simulink model "spwm"  (R2023b)
settings: Solver=VariableStepAuto  StartTime=0.0  StopTime=0.03  RelTol=1e-3
libraries: dspfdesign x1, simulink x1
settings Model: Creator=JHHK-SJM  LastModifiedBy=JHHK-SJM

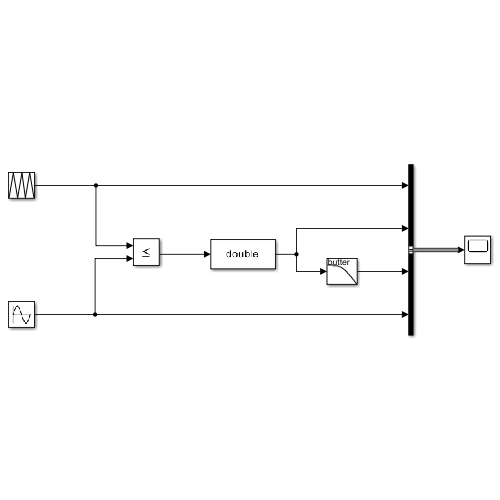
[thumbnail: Simulink's stored preview of the top-level diagram]
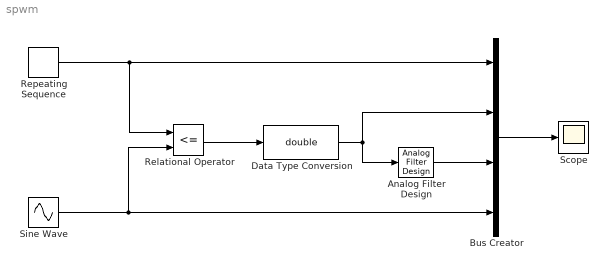
== system spwm ==
  Analog Filter Design : dspfdesign/Analog Filter Design  method=Butterworth  filttype=Lowpass  N=1  Wlo=1000*pi  Whi=80  Rp=2  Rs=40
  Bus Creator : BusCreator  Inputs=4
  Data Type Conversion : DataTypeConversion  OutDataTypeStr=double  SaturateOnIntegerOverflow=off  RndMeth=Floor
  Relational Operator : RelationalOperator  Operator=<=  OutDataTypeStr=boolean  RndMeth=Simplest  InputSameDT=off
  Repeating Sequence : simulink/Sources/Repeating Sequence  rep_seq_t=[0 2/1e4 4/1e4]  rep_seq_y=[-1 1 -1]
  Scope : Scope
  Sine Wave : Sin  Frequency=100*pi  SampleTime=0
  wires:
  Repeating Sequence/1 -> Relational Operator/1, Bus Creator/1
  Sine Wave/1 -> Relational Operator/2, Bus Creator/4
  Relational Operator/1 -> Data Type Conversion/1
  Bus Creator/1 -> Scope/1
  Data Type Conversion/1 -> Bus Creator/2, Analog Filter Design/1
  Analog Filter Design/1 -> Bus Creator/3
